simulink model "T_junction_mpc"  (R2022b)
settings: Solver=FixedStepAuto  StartTime=0.0  StopTime=293.175  FixedStep=0.025  RelTol=1e-3
values from neighbouring files (symbols this model uses):
  Aod = God.A    [mpcDesign.m]
  beta = 0.13534    [mpcDesign.m]    (also in simSysID.m)
  Bod = God.B    [mpcDesign.m]
  Cod = God.C    [mpcDesign.m]
  Dmn = Gmn.D    [mpcDesign.m]
  Dod = God.D    [mpcDesign.m]
  dt = 1/samplingRate    (= 0.025)    [plantConstants.m]    (also in sysID.m)
  eventQueue = [ ... (first row only)    [mpcDesign.m]
  forgettingFactor = 1 - dt/tau    [mpcDesign.m]
  G = idss(blkdiag(A_0, A_0),          [B_0; B_0],          blkdiag(C_0, C_0),          [D_0; D_0],          blkdiag(K_0, K_0),          x_0, dt)    [get1stOrderMdl.m]    (also in get2ndOrderMdl.m; getIntegratorMdl.m; stateEst_.m = eye(ns); stateEstimator.m = eye(ns))
  God = getoutdist(ampc)    [mpcDesign.m]
  ni = no    (= 3)    [plantConstants.m]
  no = 3    [plantConstants.m]    (also in sysID.m = length(outputs))
  np = ni + 1    [get1stOrderMdl.m]    (also in get2ndOrderMdl.m = ni + 2; getIntegratorMdl.m = ni)
  nullEv = struct('r', [0; 0; 0; 0; 0; 0], 'preT', 0, 'moveT', 0, 'postT', 0)    [mpcDesign.m]    (also in simSysID.m)
  u_max = [80; 80; 80]    [plantConstants.m]
  uwt0 = zeros(1, ni)    [mpcDesign.m]
  y_max = 612*ones(2*no, 1)    [plantConstants.m]
  ywt0 = zeros(1, 2*no)    [mpcDesign.m]    (also in simSysID.m)
undefined symbols (not defined in the file or in its folder): Discrete, lpfDen, lpfNum, N0, R0, Time, u_o, y_o
libraries: ctrlSharedLib x2, simulink_extras x1, mpclib x1
settings Model: PauseTimes=21.75  Creator=khqc  LastModifiedBy=khqc
settings DataIOCC: ExternalInput=[t, r]  OutputOption=SpecifiedOutputTimes  OutputTimes=t
settings OptimizationCC: UseDivisionForNetSlopeComputation=on  GainParamInheritBuiltInType=on  UseFloatMulNetSlope=on  StrengthReduction=on  PassReuseOutputArgsAs=Individual arguments  ZeroExternalMemoryAtStartup=off  ZeroInternalMemoryAtStartup=off  NoFixptDivByZeroProtection=on  EfficientFloat2IntCast=on  LifeSpan=1  OptimizeBlockOrder=speed  OptimizationPriority=Speed  OptimizationCustomize=off  MultiThreadedLoops=on  EfficientTunableParamExpr=on
settings DebuggingCC: ReadBeforeWriteMsg=EnableAllAsError  WriteAfterWriteMsg=EnableAllAsError  WriteAfterReadMsg=EnableAllAsError  IntegerOverflowMsg=error  ParameterTunabilityLossMsg=error  UniqueDataStoreMsg=error  BusObjectLabelMismatch=error  NonBusSignalsTreatedAsBus=error  SFInvalidInputDataAccessInChartInitDiag=error  SFTransitionOutsideNaturalParentDiag=error  SFUnreachableExecutionPathDiag=error  SFUndirectedBroadcastEventsDiag=error  IntegerSaturationMsg=error  ForceCombineOutputUpdateInSim=on
settings HardwareCC: ProdBitPerLong=64  ProdLongLongMode=on  ProdHWDeviceType=Intel->x86-64 (Linux 64)
settings ModelReferenceCC: ModelReferenceMinAlgLoopOccurrences=on
settings SFSimCC: MATLABDynamicMemAlloc=off
settings RTWCC: Description=Embedded Coder  SystemTargetFile=ert.tlc  GenCodeOnly=on  PackageGeneratedCodeAndArtifacts=on  TemplateMakefile=ert_default_tmf  GenerateReport=on  BuildConfiguration=Faster Runs  IncludeHyperlinkInReport=on  LaunchReport=on  TargetLang=C++  GenerateTraceInfo=on  GenerateTraceReport=on  GenerateTraceReportSl=on  GenerateTraceReportSf=on  GenerateTraceReportEml=on
settings CodeAppCC: ForceParamTrailComments=on  IgnoreCustomStorageClasses=off  OperatorAnnotations=on  SimulinkDataObjDesc=on  SFDataObjDesc=on  MATLABFcnDesc=on  CustomSymbolStrGlobalVar=rt$N$M  CustomSymbolStrType=$N$M  CustomSymbolStrFcn=$N$M$F  CustomSymbolStrMacro=$N$M  InsertBlockDesc=on  StateflowObjectComments=on  MATLABSourceComments=on  EnableCustomComments=on  ReqsInCode=on
settings ERTTargetCC: TargetLangStandard=C++11 (ISO)  GenerateSampleERTMain=on  CombineSignalStateStructs=on  SuppressErrorStatus=on  SupportAbsoluteTime=off  CodeInterfacePackaging=C++ class  SupportComplex=off  SupportNonInlinedSFcns=on  SupportVariableSizeSignals=on  CastingMode=Standards  RootIOFormat=Structure reference  RTWCAPIParams=on  ERTCustomFileTemplate=example_file_process.tlc  ERTFilePackagingFormat=CompactWithDataFile

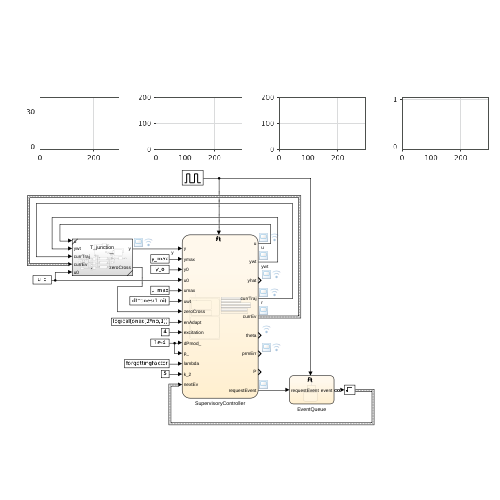
[thumbnail: Simulink's stored preview of the top-level diagram]
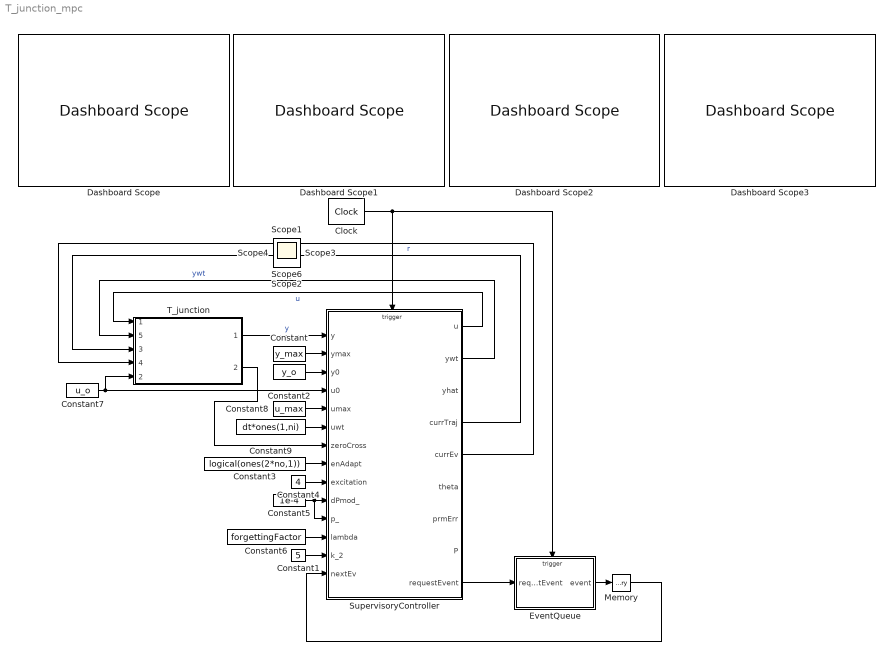
== system T_junction_mpc ==
  Clock : simulink_extras/Flip Flops/Clock  period=2*dt
  Constant : Constant  Value=y_max  VectorParams1D=off  SampleTime=-1
  Constant1 : Constant  Value=5  VectorParams1D=off  SampleTime=-1
  Constant2 : Constant  Value=y_o  VectorParams1D=off  SampleTime=-1
  Constant3 : Constant  Value=logical(ones(2*no,1))  VectorParams1D=off  SampleTime=-1
  Constant4 : Constant  Value=4  VectorParams1D=off  SampleTime=-1
  Constant5 : Constant  Value=1e-4  VectorParams1D=off  SampleTime=-1
  Constant6 : Constant  Value=forgettingFactor  VectorParams1D=off  SampleTime=-1
  Constant7 : Constant  Value=u_o  VectorParams1D=off  SampleTime=-1
  Constant8 : Constant  Value=u_max  VectorParams1D=off  SampleTime=-1
  Constant9 : Constant  Value=dt*ones(1,ni)  VectorParams1D=off  SampleTime=-1
  Dashboard Scope{,1..3} (4 alike) : DashboardScope  Ymin=0  Ymax=200
  EventQueue : Stateflow chart  TreatAsAtomicUnit=on
  Memory : Memory  InitialCondition=nullEv
  SupervisoryController : Stateflow chart  TreatAsAtomicUnit=on
  T_junction : Subsystem  ReferencedSubsystem=T_junction
      settings: PortSchema="{\"entries\":[{\"content\":{\"sides\":[{\"content\":{\"connectorIds\":[\"In1\",\"In5\",\"In3\",\"In4\",\"In2\"]},\"type\":\"ConnectorPlacement.EquallySpacedRectSide\",\"uuid\":\"0943685f-600e-41af-a665-bcc16d9a094a\"},{\"content\":{\"connectorIds\":[\"Out1\",\"Out2\"],\"side\":\"RIGHT\"},\"type\":\"ConnectorPlacement.EquallySpacedRectSide\",\"uuid\":\"88ff40b9-19c0-4ac1-b133-2a32304c8b0f\"},{\"content\":{\"connectorIds\":[],\"side\":\"TOP\"},\"type\":\"ConnectorPlacement.EquallySpacedRectSide\",\"uuid\":\"62f73c3a-6759-48ef-88af-8d02c7b37c1f\"}]},\"type\":\"ConnectorPlacement.EquallySpacedConnector\",\"uuid\":\"9de5309d-a658-4a97-a42e-d25e12f93191\"}],\"packageUris\":[\"http://schema.mathworks.com/mf0/Connector/R2020b\"],\"version\":\"1.0\"}"
  Scope{,1..4,6} (6 alike) : Scope
  wires:
  SupervisoryController/1(u) -> T_junction/1  "u"
  Clock/1 -> EventQueue/Trigger, SupervisoryController/Trigger
  Constant/1 -> SupervisoryController/2(ymax)
  Constant7/1 -> SupervisoryController/4(u0), T_junction/2
  Constant3/1 -> SupervisoryController/8(enAdapt)
  T_junction/1 -> SupervisoryController/1(y)  "y"
  Constant4/1 -> SupervisoryController/9(excitation)
  Constant2/1 -> SupervisoryController/3(y0)
  Memory/1 -> SupervisoryController/14(nextEv)
  EventQueue/1(event) -> Memory/1
  Constant5/1 -> SupervisoryController/10(dPmod_), SupervisoryController/11(p_)
  Constant6/1 -> SupervisoryController/12(lambda)
  SupervisoryController/9(requestEvent) -> EventQueue/1(requestEvent)
  SupervisoryController/5(currEv) -> T_junction/4
  SupervisoryController/4(currTraj) -> T_junction/3  "r"
  SupervisoryController/2(ywt) -> T_junction/5  "ywt"
  T_junction/2 -> SupervisoryController/7(zeroCross)
  Constant1/1 -> SupervisoryController/13(k_2)
  Constant8/1 -> SupervisoryController/5(umax)
  Constant9/1 -> SupervisoryController/6(uwt)

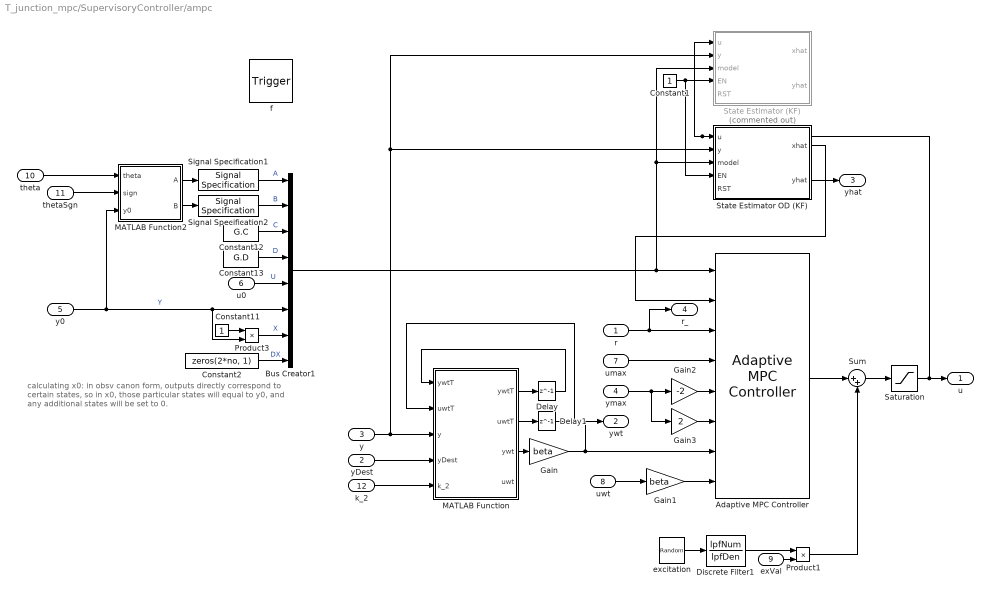
== system T_junction_mpc/SupervisoryController/ampc ==
  note: calculating x0:
      | in obsv canon form, outputs directly correspond to certain states, so in x0, those particular states will equal to y0, and any additional states will be set to 0.
  r : Inport  OutDataTypeStr=double  PortDimensions=[2*no, 1]
  yDest : Inport  Port=2  OutDataTypeStr=double  PortDimensions=[2*no, 1]
  y : Inport  Port=3  OutDataTypeStr=double  PortDimensions=[2*no, 1]
  ymax : Inport  Port=4  OutDataTypeStr=double  PortDimensions=[2*no,1]
  y0 : Inport  Port=5  OutDataTypeStr=double  PortDimensions=[2*no, 1]
  u0 : Inport  Port=6  OutDataTypeStr=double  PortDimensions=[ni, 1]
  umax : Inport  Port=7  OutDataTypeStr=double  PortDimensions=[ni, 1]
  uwt : Inport  Port=8  OutDataTypeStr=double  PortDimensions=[1, ni]
  exVal : Inport  Port=9  OutDataTypeStr=double  PortDimensions=1
  theta : Inport  Port=10  OutDataTypeStr=double  PortDimensions=[2*np*no, 1]
  thetaSgn : Inport  Port=11  OutDataTypeStr=double  PortDimensions=[2*np*no, 1]
  k_2 : Inport  Port=12  OutDataTypeStr=double  PortDimensions=1
  f : TriggerPort  TriggerType=function-call  VariantControl=(inherit)
      settings: CopyFcn=Stateflow.SLINSF.SimulinkMan.removeBlockPreDeleteFcn  PreDeleteFcn=Stateflow.SLINSF.SimulinkMan.unsafePredeleteFcn
  Adaptive MPC Controller : mpclib/Adaptive MPC Controller  SCDEnableBlockLinearizationSpecification=on  mpcobj=ampc  enable_value=0  updateMPCinCallerWorkspace=on  md_inport=off  mv_inport=off  uref_inport=off  return_cost=off  return_mvseq=off  return_qpstatus=off  return_xseq=off  return_state=off  return_ovseq=off  state_inport=on  isltv_plant=off  umin_inport=off  umax_inport=on  ymin_inport=on  ymax_inport=on  cc_inport=off  ywt_inport=on  uwt_inport=on  duwt_inport=off  rhoeps_inport=off  pm_inport=off  MaximumP=10  HorizonChoice=FixedHorizon  BlockDataType=double  SampleTimeInherited=on  switch_inport=off
  Bus Creator1 : BusCreator  Inputs=8  OutDataTypeStr=Bus: mdl_bus  NonVirtualBus=on
  Constant1 : Constant  VectorParams1D=off
  Constant11 : Constant  VectorParams1D=off
  Constant12 : Constant  Value=G.C  VectorParams1D=off
  Constant13 : Constant  Value=G.D  VectorParams1D=off
  Constant2 : Constant  Value=zeros(2*no, 1)  VectorParams1D=off
  Delay : Delay  DelayLength=1  InitialCondition=ywt0
  Delay1 : Delay  DelayLength=1  InitialCondition=uwt0
  Discrete Filter1 : DiscreteFilter  Numerator=lpfNum  Denominator=lpfDen
  Gain : Gain  Gain=beta
  Gain1 : Gain  Gain=beta
  Gain2 : Gain  Gain=-2
  Gain3 : Gain  Gain=2
  MATLAB Function : MATLAB Function  TreatAsAtomicUnit=on
  MATLAB Function2 : MATLAB Function  TreatAsAtomicUnit=on
  Product1 : Product
  Product3 : Product
  Saturation : Saturate  UpperLimit=1000  LowerLimit=0
  Signal Specification1 : SignalSpecification  Dimensions=size(G.A)
  Signal Specification2 : SignalSpecification  Dimensions=size(G.B)
  State Estimator (KF) : Subsystem  Commented=on
      settings: MinAlgLoopOccurrences=on
  State Estimator OD (KF) : Subsystem
      settings: MinAlgLoopOccurrences=on
  Sum : Sum  Inputs=|++
  excitation : RandomNumber  Mean=[0 0 0]  Variance=[1 1 1]  Seed=[12345 12346 12347]
  u : Outport
  ywt : Outport  Port=2
  yhat : Outport  Port=3
  r_ : Outport  Port=4
  wires:
  Saturation/1 -> u/1, State Estimator (KF)/1(u), State Estimator OD (KF)/1(u)
  excitation/1 -> Discrete Filter1/1
  Discrete Filter1/1 -> Product1/1
  exVal/1 -> Product1/2
  Product1/1 -> Sum/2
  Adaptive MPC Controller/1 -> Sum/1
  r/1 -> r_/1, Adaptive MPC Controller/3
  Delay/1 -> MATLAB Function/1("ywtT ")
  ymax/1 -> Gain3/1, Gain2/1
  MATLAB Function/1(ywtT) -> Delay/1
  MATLAB Function/2(uwtT) -> Delay1/1
  Delay1/1 -> MATLAB Function/2("uwtT ")
  Gain/1 -> Adaptive MPC Controller/7, ywt/1
  Gain1/1 -> Adaptive MPC Controller/8
  Sum/1 -> Saturation/1
  uwt/1 -> Gain1/1
  MATLAB Function/3(ywt) -> Gain/1
  Gain2/1 -> Adaptive MPC Controller/5
  yDest/1 -> MATLAB Function/4(yDest)
  Bus Creator1/1 -> State Estimator (KF)/3(model), State Estimator OD (KF)/3(model), Adaptive MPC Controller/1
  Product3/1 -> Bus Creator1/7  "X"
  Signal Specification1/1 -> Bus Creator1/1  "A"
  Constant11/1 -> Product3/1
  y0/1 -> MATLAB Function2/3(y0), Product3/2, Bus Creator1/6  "Y"
  Constant13/1 -> Bus Creator1/4  "D"
  Constant12/1 -> Bus Creator1/3  "C"
  MATLAB Function2/2(B) -> Signal Specification2/1
  MATLAB Function2/1(A) -> Signal Specification1/1
  Signal Specification2/1 -> Bus Creator1/2  "B"
  Constant2/1 -> Bus Creator1/8  "DX"
  thetaSgn/1 -> MATLAB Function2/2(sign)
  theta/1 -> MATLAB Function2/1(theta)
  u0/1 -> Bus Creator1/5  "U"
  Constant1/1 -> State Estimator OD (KF)/4(EN), State Estimator (KF)/4(EN)
  Gain3/1 -> Adaptive MPC Controller/6
  y/1 -> State Estimator (KF)/2(y), State Estimator OD (KF)/2(y), MATLAB Function/3(y)
  State Estimator OD (KF)/2(yhat) -> yhat/1
  State Estimator OD (KF)/1(xhat) -> Adaptive MPC Controller/2
  k_2/1 -> MATLAB Function/5(k_2)
  umax/1 -> Adaptive MPC Controller/4

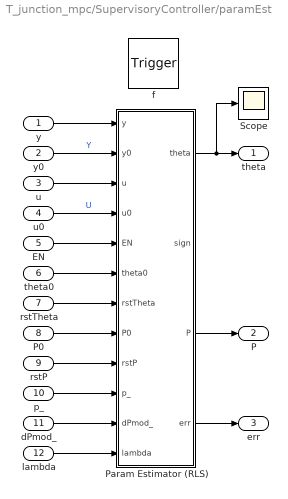
== system T_junction_mpc/SupervisoryController/paramEst ==
  y : Inport  OutDataTypeStr=double  PortDimensions=[no, 1]
  y0 : Inport  Port=2  OutDataTypeStr=double  PortDimensions=[no, 1]
  u : Inport  Port=3  OutDataTypeStr=double  PortDimensions=[ni, 1]
  u0 : Inport  Port=4  OutDataTypeStr=double  PortDimensions=[ni, 1]
  EN : Inport  Port=5  OutDataTypeStr=boolean  PortDimensions=[no, 1]
  theta0 : Inport  Port=6  OutDataTypeStr=double  PortDimensions=[np*no, 1]
  rstTheta : Inport  Port=7  OutDataTypeStr=boolean  PortDimensions=1
  P0 : Inport  Port=8  OutDataTypeStr=double  PortDimensions=[np*no, np*no]
  rstP : Inport  Port=9  OutDataTypeStr=boolean  PortDimensions=1
  p_ : Inport  Port=10  OutDataTypeStr=double  PortDimensions=1
  dPmod_ : Inport  Port=11  OutDataTypeStr=double  PortDimensions=1
  lambda : Inport  Port=12  OutDataTypeStr=double  PortDimensions=1
  f : TriggerPort  TriggerType=function-call  VariantControl=(inherit)
      settings: CopyFcn=Stateflow.SLINSF.SimulinkMan.removeBlockPreDeleteFcn  PreDeleteFcn=Stateflow.SLINSF.SimulinkMan.unsafePredeleteFcn
  Param Estimator (RLS) : Subsystem
  Scope : Scope
  theta : Outport
  P : Outport  Port=2
  err : Outport  Port=3
  wires:
  y0/1 -> Param Estimator (RLS)/2(y0)  "Y"
  u0/1 -> Param Estimator (RLS)/4(u0)  "U"
  y/1 -> Param Estimator (RLS)/1(y)
  u/1 -> Param Estimator (RLS)/3(u)
  EN/1 -> Param Estimator (RLS)/5(EN)
  theta0/1 -> Param Estimator (RLS)/6(theta0)
  rstTheta/1 -> Param Estimator (RLS)/7(rstTheta)
  P0/1 -> Param Estimator (RLS)/8(P0)
  rstP/1 -> Param Estimator (RLS)/9(rstP)
  p_/1 -> Param Estimator (RLS)/10(p_)
  dPmod_/1 -> Param Estimator (RLS)/11(dPmod_)
  lambda/1 -> Param Estimator (RLS)/12(lambda)
  Param Estimator (RLS)/1(theta) -> Scope/1, theta/1
  Param Estimator (RLS)/3(P) -> P/1
  Param Estimator (RLS)/4(err) -> err/1

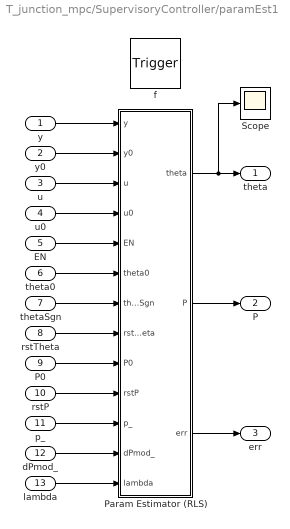
== system T_junction_mpc/SupervisoryController/paramEst1 ==
  y : Inport  OutDataTypeStr=double  PortDimensions=[no, 1]
  y0 : Inport  Port=2  OutDataTypeStr=double  PortDimensions=[no, 1]
  u : Inport  Port=3  OutDataTypeStr=double  PortDimensions=[ni, 1]
  u0 : Inport  Port=4  OutDataTypeStr=double  PortDimensions=[ni, 1]
  EN : Inport  Port=5  OutDataTypeStr=boolean  PortDimensions=[no, 1]
  theta0 : Inport  Port=6  OutDataTypeStr=double  PortDimensions=[np*no, 1]
  thetaSgn : Inport  Port=7  OutDataTypeStr=double  PortDimensions=[np*no, 1]
  rstTheta : Inport  Port=8  OutDataTypeStr=boolean  PortDimensions=1
  P0 : Inport  Port=9  OutDataTypeStr=double  PortDimensions=[np*no, np*no]
  rstP : Inport  Port=10  OutDataTypeStr=boolean  PortDimensions=1
  p_ : Inport  Port=11  OutDataTypeStr=double  PortDimensions=1
  dPmod_ : Inport  Port=12  OutDataTypeStr=double  PortDimensions=1
  lambda : Inport  Port=13  OutDataTypeStr=double  PortDimensions=1
  f : TriggerPort  TriggerType=function-call  VariantControl=(inherit)
      settings: CopyFcn=Stateflow.SLINSF.SimulinkMan.removeBlockPreDeleteFcn  PreDeleteFcn=Stateflow.SLINSF.SimulinkMan.unsafePredeleteFcn
  Param Estimator (RLS) : Subsystem
  Scope : Scope
  theta : Outport
  P : Outport  Port=2
  err : Outport  Port=3
  wires:
  y0/1 -> Param Estimator (RLS)/2(y0)
  u0/1 -> Param Estimator (RLS)/4(u0)
  y/1 -> Param Estimator (RLS)/1(y)
  u/1 -> Param Estimator (RLS)/3(u)
  EN/1 -> Param Estimator (RLS)/5(EN)
  theta0/1 -> Param Estimator (RLS)/6(theta0)
  rstTheta/1 -> Param Estimator (RLS)/8(rstTheta)
  P0/1 -> Param Estimator (RLS)/9(P0)
  rstP/1 -> Param Estimator (RLS)/10(rstP)
  p_/1 -> Param Estimator (RLS)/11(p_)
  dPmod_/1 -> Param Estimator (RLS)/12(dPmod_)
  lambda/1 -> Param Estimator (RLS)/13(lambda)
  Param Estimator (RLS)/1(theta) -> Scope/1, theta/1
  Param Estimator (RLS)/2(P) -> P/1
  Param Estimator (RLS)/3(err) -> err/1
  thetaSgn/1 -> Param Estimator (RLS)/7(thetaSgn)

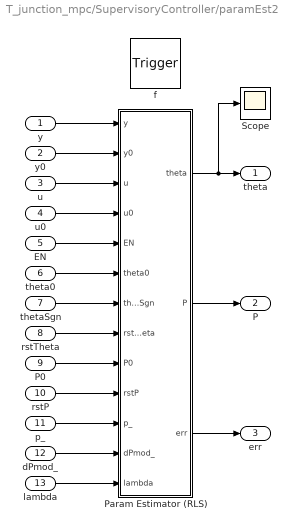
== system T_junction_mpc/SupervisoryController/paramEst2 ==
  y : Inport  OutDataTypeStr=double  PortDimensions=[no, 1]
  y0 : Inport  Port=2  OutDataTypeStr=double  PortDimensions=[no, 1]
  u : Inport  Port=3  OutDataTypeStr=double  PortDimensions=[ni, 1]
  u0 : Inport  Port=4  OutDataTypeStr=double  PortDimensions=[ni, 1]
  EN : Inport  Port=5  OutDataTypeStr=boolean  PortDimensions=[no, 1]
  theta0 : Inport  Port=6  OutDataTypeStr=double  PortDimensions=[np*no, 1]
  thetaSgn : Inport  Port=7  OutDataTypeStr=double  PortDimensions=[np*no, 1]
  rstTheta : Inport  Port=8  OutDataTypeStr=boolean  PortDimensions=1
  P0 : Inport  Port=9  OutDataTypeStr=double  PortDimensions=[np*no, np*no]
  rstP : Inport  Port=10  OutDataTypeStr=boolean  PortDimensions=1
  p_ : Inport  Port=11  OutDataTypeStr=double  PortDimensions=1
  dPmod_ : Inport  Port=12  OutDataTypeStr=double  PortDimensions=1
  lambda : Inport  Port=13  OutDataTypeStr=double  PortDimensions=1
  f : TriggerPort  TriggerType=function-call  VariantControl=(inherit)
      settings: CopyFcn=Stateflow.SLINSF.SimulinkMan.removeBlockPreDeleteFcn  PreDeleteFcn=Stateflow.SLINSF.SimulinkMan.unsafePredeleteFcn
  Param Estimator (RLS) : Subsystem
  Scope : Scope
  theta : Outport
  P : Outport  Port=2
  err : Outport  Port=3
  wires:
  y0/1 -> Param Estimator (RLS)/2(y0)
  u0/1 -> Param Estimator (RLS)/4(u0)
  y/1 -> Param Estimator (RLS)/1(y)
  u/1 -> Param Estimator (RLS)/3(u)
  EN/1 -> Param Estimator (RLS)/5(EN)
  theta0/1 -> Param Estimator (RLS)/6(theta0)
  rstTheta/1 -> Param Estimator (RLS)/8(rstTheta)
  P0/1 -> Param Estimator (RLS)/9(P0)
  rstP/1 -> Param Estimator (RLS)/10(rstP)
  p_/1 -> Param Estimator (RLS)/11(p_)
  dPmod_/1 -> Param Estimator (RLS)/12(dPmod_)
  lambda/1 -> Param Estimator (RLS)/13(lambda)
  Param Estimator (RLS)/1(theta) -> Scope/1, theta/1
  Param Estimator (RLS)/2(P) -> P/1
  Param Estimator (RLS)/3(err) -> err/1
  thetaSgn/1 -> Param Estimator (RLS)/7(thetaSgn)

== system T_junction_mpc/SupervisoryController/ampc/State Estimator (KF) ==
  u : Inport
  y : Inport  Port=2
  model : Inport  Port=3
  EN : Inport  Port=4
  RST : Inport  Port=5  PortDimensions=1
  Bus Selector : BusSelector  OutputSignals=A,B,C,D,U,Y,X,DX
  Display : Display
  Display1 : Display
  Kalman Filter2 : ctrlSharedLib/Kalman Filter  TimeDomain=Discrete-Time  UseCurrentEstimator=off  ModelSource=Input port  ModelSourceVariable=ss(0.95,1,1,0,1)  A=0.95  B=1  C=1  D=0  NumberOfStates=size(G.A,1)  NumberOfInputs=size(G.B,2)  NumberOfOutputs=size(G.C,1)  InitialEstimateSource=Dialog  X0=zeros(size(G.A,1),1)  P0=eye(size(G.A,1))  UseK=off  UseGH=off  NumberOfProcessNoiseInputs=1  G=eye(2)  TimeInvariantG=on  H=zeros(1,2)  TimeInvariantH=on  Q=Q0  TimeInvariantQ=off  R=R0  TimeInvariantR=off  N=N0  TimeInvariantN=off  AddInputPort=on  AddEnablePort=on  ExternalReset=Level  OutputEstimatedY=on  OutputP=off  Ts=-1
  MATLAB Function : MATLAB Function  TreatAsAtomicUnit=on
  Sum1 : Sum  Inputs=|+-
  Sum2 : Sum  Inputs=|++
  Sum3 : Sum  Inputs=|++
  Sum6 : Sum  Inputs=|+-
  xhat : Outport
  yhat : Outport  Port=2
  wires:
  Kalman Filter2/1 -> Sum2/1
  MATLAB Function/5(Q) -> Kalman Filter2/9
  MATLAB Function/2(B) -> Display1/1, Kalman Filter2/6
  RST/1 -> Kalman Filter2/4
  MATLAB Function/1(A) -> Display/1, Kalman Filter2/5
  model/1 -> Bus Selector/1
  Bus Selector/7 -> Sum2/2  "<X>"
  MATLAB Function/3(C) -> Kalman Filter2/7
  Bus Selector/1 -> MATLAB Function/1(Ap)  "<A>"
  Bus Selector/2 -> MATLAB Function/2(Bp)  "<B>"
  MATLAB Function/4(D) -> Kalman Filter2/8
  EN/1 -> Kalman Filter2/3
  Bus Selector/3 -> MATLAB Function/3(Cp)  "<C>"
  Bus Selector/4 -> MATLAB Function/4(Dp)  "<D>"
  Bus Selector/5 -> Sum1/2  "<U>"
  Sum2/1 -> xhat/1
  Bus Selector/6 -> Sum3/2, Sum6/2  "<Y>"
  y/1 -> Sum6/1
  MATLAB Function/6(R) -> Kalman Filter2/10
  MATLAB Function/7(N) -> Kalman Filter2/11
  u/1 -> Sum1/1
  Sum1/1 -> Kalman Filter2/1
  Sum6/1 -> Kalman Filter2/2
  Kalman Filter2/2 -> Sum3/1
  Sum3/1 -> yhat/1

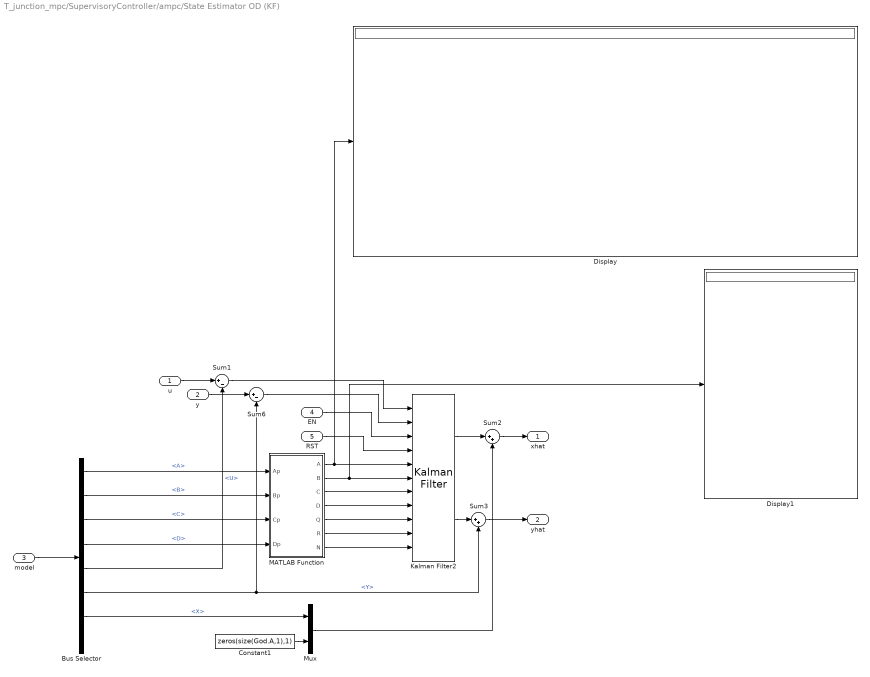
== system T_junction_mpc/SupervisoryController/ampc/State Estimator OD (KF) ==
  u : Inport
  y : Inport  Port=2
  model : Inport  Port=3
  EN : Inport  Port=4
  RST : Inport  Port=5  PortDimensions=1
  Bus Selector : BusSelector  OutputSignals=A,B,C,D,U,Y,X,DX
  Constant1 : Constant  Value=zeros(size(God.A,1),1)  VectorParams1D=off
  Display : Display
  Display1 : Display
  Kalman Filter2 : ctrlSharedLib/Kalman Filter  TimeDomain=Discrete-Time  UseCurrentEstimator=off  ModelSource=Input port  ModelSourceVariable=ss(0.95,1,1,0,1)  A=0.95  B=1  C=1  D=0  NumberOfStates=size(G.A,1) + size(God.A,1)  NumberOfInputs=size(G.B,2)  NumberOfOutputs=size(G.C,1)  InitialEstimateSource=Dialog  X0=zeros(size(G.A,1) + size(God.A,1),1)  P0=eye(size(G.A,1) + size(God.A,1))  UseK=off  UseGH=off  NumberOfProcessNoiseInputs=1  G=eye(2)  TimeInvariantG=on  H=zeros(1,2)  TimeInvariantH=on  Q=Q0  TimeInvariantQ=off  R=R0  TimeInvariantR=off  N=N0  TimeInvariantN=off  AddInputPort=on  AddEnablePort=on  ExternalReset=Level  OutputEstimatedY=on  OutputP=off  Ts=-1
  MATLAB Function : MATLAB Function  TreatAsAtomicUnit=on
  Mux : Mux  Inputs=2
  Sum1 : Sum  Inputs=|+-
  Sum2 : Sum  Inputs=|++
  Sum3 : Sum  Inputs=|++
  Sum6 : Sum  Inputs=|+-
  xhat : Outport
  yhat : Outport  Port=2
  wires:
  Kalman Filter2/1 -> Sum2/1
  MATLAB Function/5(Q) -> Kalman Filter2/9
  MATLAB Function/2(B) -> Display1/1, Kalman Filter2/6
  RST/1 -> Kalman Filter2/4
  MATLAB Function/1(A) -> Display/1, Kalman Filter2/5
  model/1 -> Bus Selector/1
  Bus Selector/7 -> Mux/1  "<X>"
  MATLAB Function/3(C) -> Kalman Filter2/7
  Bus Selector/1 -> MATLAB Function/1(Ap)  "<A>"
  Bus Selector/2 -> MATLAB Function/2(Bp)  "<B>"
  MATLAB Function/4(D) -> Kalman Filter2/8
  EN/1 -> Kalman Filter2/3
  Bus Selector/3 -> MATLAB Function/3(Cp)  "<C>"
  Bus Selector/4 -> MATLAB Function/4(Dp)  "<D>"
  Constant1/1 -> Mux/2
  Bus Selector/5 -> Sum1/2  "<U>"
  Sum2/1 -> xhat/1
  Bus Selector/6 -> Sum3/2, Sum6/2  "<Y>"
  y/1 -> Sum6/1
  MATLAB Function/6(R) -> Kalman Filter2/10
  MATLAB Function/7(N) -> Kalman Filter2/11
  u/1 -> Sum1/1
  Sum1/1 -> Kalman Filter2/1
  Sum6/1 -> Kalman Filter2/2
  Kalman Filter2/2 -> Sum3/1
  Sum3/1 -> yhat/1
  Mux/1 -> Sum2/2

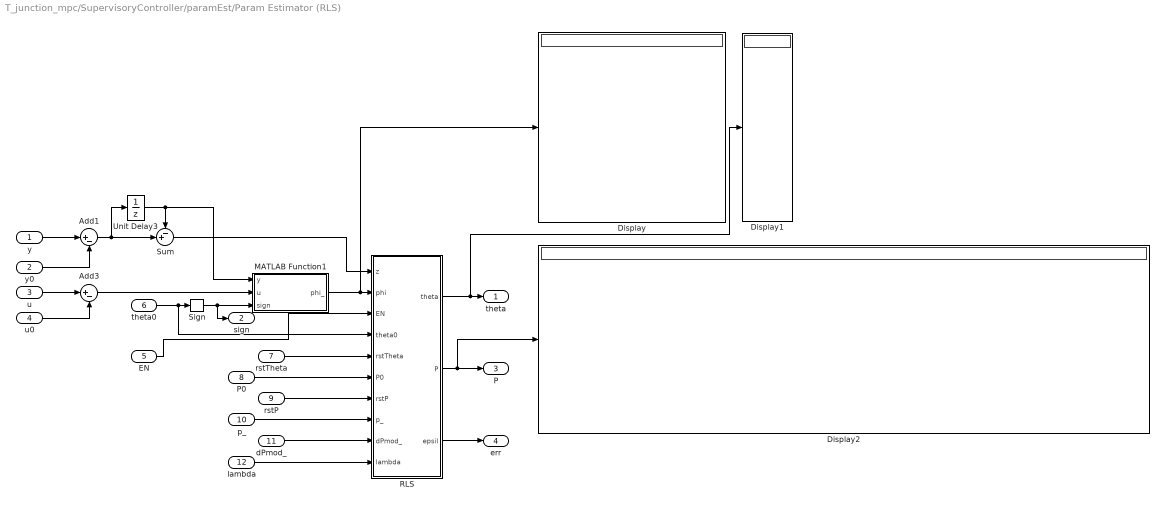
== system T_junction_mpc/SupervisoryController/paramEst/Param Estimator (RLS) ==
  y : Inport
  y0 : Inport  Port=2
  u : Inport  Port=3
  u0 : Inport  Port=4
  EN : Inport  Port=5
  theta0 : Inport  Port=6
  rstTheta : Inport  Port=7
  P0 : Inport  Port=8
  rstP : Inport  Port=9
  p_ : Inport  Port=10
  dPmod_ : Inport  Port=11
  lambda : Inport  Port=12
  Add1 : Sum  Inputs=|+-
  Add3 : Sum  Inputs=|+-
  Display : Display
  Display1 : Display
  Display2 : Display
  MATLAB Function1 : MATLAB Function  TreatAsAtomicUnit=on
  RLS : Subsystem
  Sign : Signum
  Sum : Sum  Inputs=-+|
  Unit Delay3 : UnitDelay  SampleTime=-1  HasFrameUpgradeWarning=on
  theta : Outport
  sign : Outport  Port=2
  P : Outport  Port=3
  err : Outport  Port=4
  wires:
  p_/1 -> RLS/8(p_)
  P0/1 -> RLS/6(P0)
  RLS/3(epsil) -> err/1
  u/1 -> Add3/1
  Sign/1 -> sign/1, MATLAB Function1/3(sign)
  Sum/1 -> RLS/1(z)
  rstTheta/1 -> RLS/5(rstTheta)
  Add1/1 -> Sum/2, Unit Delay3/1
  y0/1 -> Add1/2
  theta0/1 -> RLS/4(theta0), Sign/1
  y/1 -> Add1/1
  dPmod_/1 -> RLS/9(dPmod_)
  Add3/1 -> MATLAB Function1/2(u)
  Unit Delay3/1 -> MATLAB Function1/1(y), Sum/1
  RLS/1(theta) -> theta/1, Display1/1
  lambda/1 -> RLS/10(lambda)
  rstP/1 -> RLS/7(rstP)
  RLS/2(P) -> P/1, Display2/1
  MATLAB Function1/1(phi_) -> Display/1, RLS/2(phi)
  u0/1 -> Add3/2
  EN/1 -> RLS/3(EN)

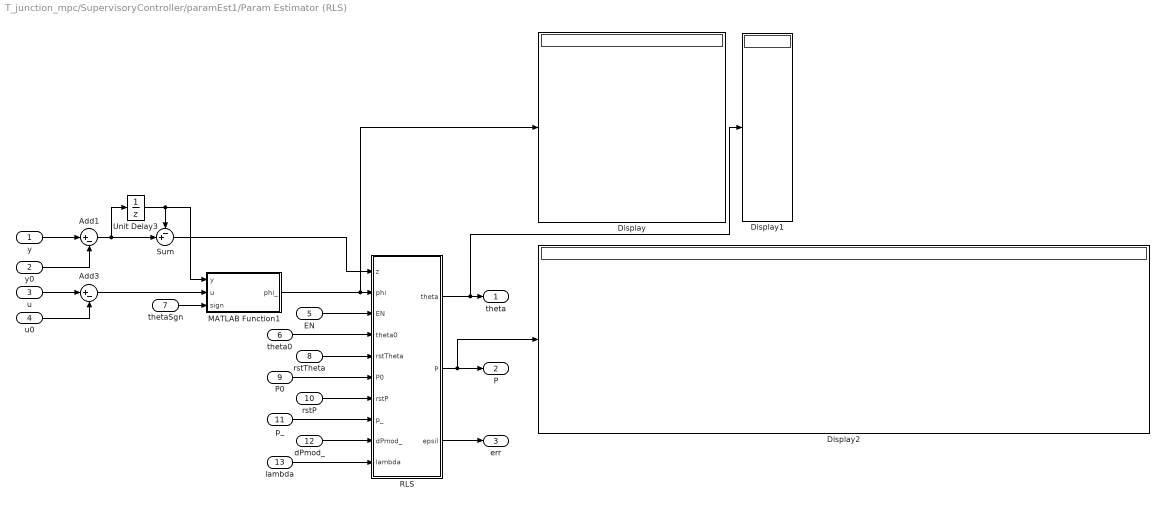
== system T_junction_mpc/SupervisoryController/paramEst1/Param Estimator (RLS) ==
  y : Inport
  y0 : Inport  Port=2
  u : Inport  Port=3
  u0 : Inport  Port=4
  EN : Inport  Port=5
  theta0 : Inport  Port=6
  thetaSgn : Inport  Port=7
  rstTheta : Inport  Port=8
  P0 : Inport  Port=9
  rstP : Inport  Port=10
  p_ : Inport  Port=11
  dPmod_ : Inport  Port=12
  lambda : Inport  Port=13
  Add1 : Sum  Inputs=|+-
  Add3 : Sum  Inputs=|+-
  Display : Display
  Display1 : Display
  Display2 : Display
  MATLAB Function1 : MATLAB Function  TreatAsAtomicUnit=on
  RLS : Subsystem
  Sum : Sum  Inputs=-+|
  Unit Delay3 : UnitDelay  SampleTime=-1  HasFrameUpgradeWarning=on
  theta : Outport
  P : Outport  Port=2
  err : Outport  Port=3
  wires:
  p_/1 -> RLS/8(p_)
  P0/1 -> RLS/6(P0)
  RLS/3(epsil) -> err/1
  u/1 -> Add3/1
  thetaSgn/1 -> MATLAB Function1/3(sign)
  Sum/1 -> RLS/1(z)
  rstTheta/1 -> RLS/5(rstTheta)
  Add1/1 -> Sum/2, Unit Delay3/1
  y0/1 -> Add1/2
  theta0/1 -> RLS/4(theta0)
  y/1 -> Add1/1
  dPmod_/1 -> RLS/9(dPmod_)
  Add3/1 -> MATLAB Function1/2(u)
  Unit Delay3/1 -> MATLAB Function1/1(y), Sum/1
  RLS/1(theta) -> theta/1, Display1/1
  lambda/1 -> RLS/10(lambda)
  rstP/1 -> RLS/7(rstP)
  RLS/2(P) -> P/1, Display2/1
  MATLAB Function1/1(phi_) -> Display/1, RLS/2(phi)
  u0/1 -> Add3/2
  EN/1 -> RLS/3(EN)

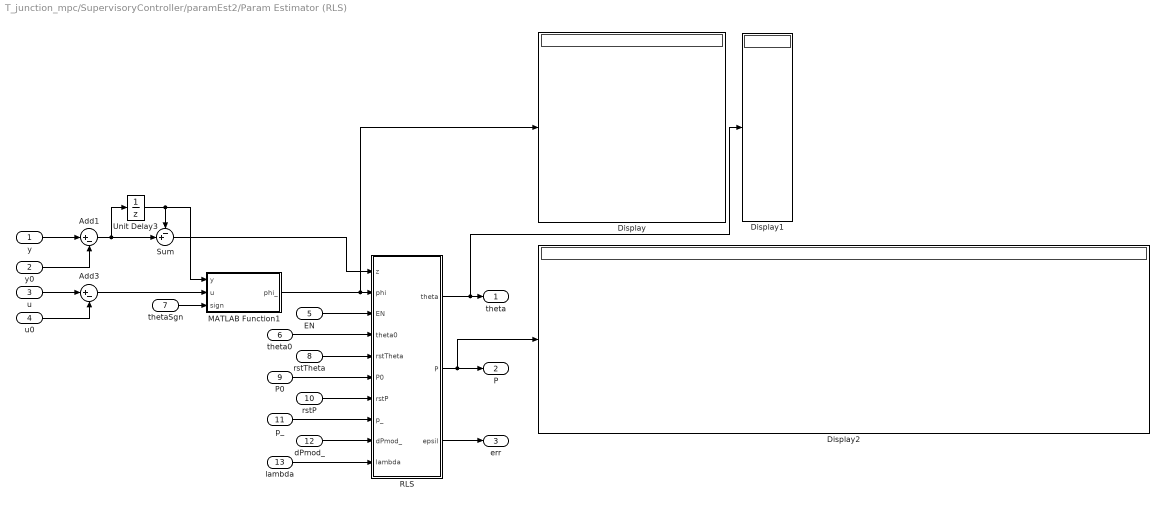
== system T_junction_mpc/SupervisoryController/paramEst2/Param Estimator (RLS) ==
  y : Inport
  y0 : Inport  Port=2
  u : Inport  Port=3
  u0 : Inport  Port=4
  EN : Inport  Port=5
  theta0 : Inport  Port=6
  thetaSgn : Inport  Port=7
  rstTheta : Inport  Port=8
  P0 : Inport  Port=9
  rstP : Inport  Port=10
  p_ : Inport  Port=11
  dPmod_ : Inport  Port=12
  lambda : Inport  Port=13
  Add1 : Sum  Inputs=|+-
  Add3 : Sum  Inputs=|+-
  Display : Display
  Display1 : Display
  Display2 : Display
  MATLAB Function1 : MATLAB Function  TreatAsAtomicUnit=on
  RLS : Subsystem
  Sum : Sum  Inputs=-+|
  Unit Delay3 : UnitDelay  SampleTime=-1  HasFrameUpgradeWarning=on
  theta : Outport
  P : Outport  Port=2
  err : Outport  Port=3
  wires:
  p_/1 -> RLS/8(p_)
  P0/1 -> RLS/6(P0)
  RLS/3(epsil) -> err/1
  u/1 -> Add3/1
  thetaSgn/1 -> MATLAB Function1/3(sign)
  Sum/1 -> RLS/1(z)
  rstTheta/1 -> RLS/5(rstTheta)
  Add1/1 -> Sum/2, Unit Delay3/1
  y0/1 -> Add1/2
  theta0/1 -> RLS/4(theta0)
  y/1 -> Add1/1
  dPmod_/1 -> RLS/9(dPmod_)
  Add3/1 -> MATLAB Function1/2(u)
  Unit Delay3/1 -> MATLAB Function1/1(y), Sum/1
  RLS/1(theta) -> theta/1, Display1/1
  lambda/1 -> RLS/10(lambda)
  rstP/1 -> RLS/7(rstP)
  RLS/2(P) -> P/1, Display2/1
  MATLAB Function1/1(phi_) -> Display/1, RLS/2(phi)
  u0/1 -> Add3/2
  EN/1 -> RLS/3(EN)

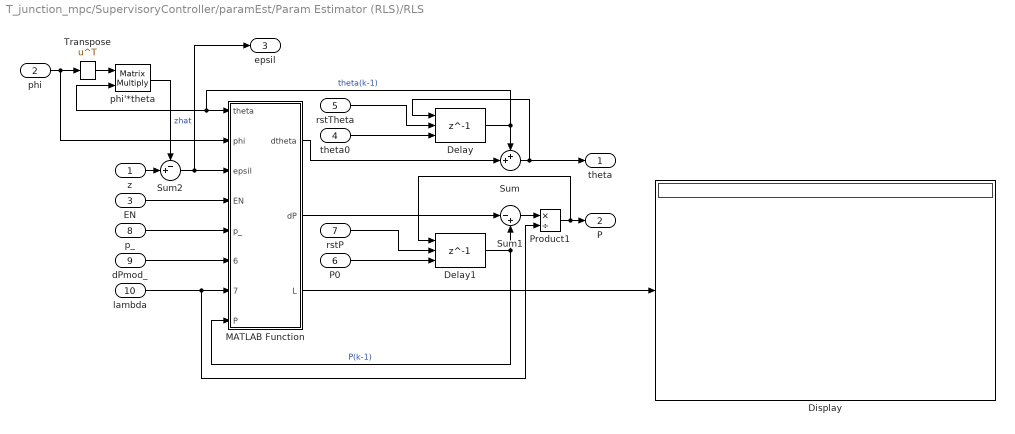
== system T_junction_mpc/SupervisoryController/paramEst/Param Estimator (RLS)/RLS ==
  z : Inport
  phi : Inport  Port=2
  EN : Inport  Port=3
  theta0 : Inport  Port=4
  rstTheta : Inport  Port=5
  P0 : Inport  Port=6
  rstP : Inport  Port=7
  p_ : Inport  Port=8
  dPmod_ : Inport  Port=9
  lambda : Inport  Port=10
  Delay : Delay  DelayLength=1  InitialConditionSource=Input port  ExternalReset=Rising
      settings: InputPortMap=u0,r5,p4
  Delay1 : Delay  DelayLength=1  InitialConditionSource=Input port  ExternalReset=Rising
      settings: InputPortMap=u0,r5,p4
  Display : Display
  MATLAB Function : MATLAB Function  TreatAsAtomicUnit=on
  Product1 : Product  Inputs=*/
  Sum : Sum  Inputs=++|
  Sum1 : Sum  Inputs=|-+
  Sum2 : Sum  Inputs=-+|
  Transpose : Math  Operator=transpose
  phi'*theta : Product  Multiplication=Matrix(*)
  theta : Outport
  P : Outport  Port=2
  epsil : Outport  Port=3
  wires:
  phi/1 -> MATLAB Function/2(phi), Transpose/1
  EN/1 -> MATLAB Function/4(EN)
  P0/1 -> Delay1/3
  MATLAB Function/1(dtheta) -> Sum/2
  Delay/1 -> Sum/1, phi'*theta/2, MATLAB Function/1(theta)  "theta(k-1)"
  Sum/1 -> theta/1, Delay/1
  MATLAB Function/2(dP) -> Sum1/1
  Sum1/1 -> Product1/1
  Delay1/1 -> Sum1/2, MATLAB Function/8(P)  "P(k-1)"
  Product1/1 -> Delay1/1, P/1
  z/1 -> Sum2/2
  Transpose/1 -> phi'*theta/1
  phi'*theta/1 -> Sum2/1  "zhat"
  Sum2/1 -> epsil/1, MATLAB Function/3(epsil)
  theta0/1 -> Delay/3
  dPmod_/1 -> MATLAB Function/6(dPmod_)
  p_/1 -> MATLAB Function/5(p_)
  rstTheta/1 -> Delay/2
  rstP/1 -> Delay1/2
  lambda/1 -> Product1/2, MATLAB Function/7(lambda)
  MATLAB Function/3(L) -> Display/1

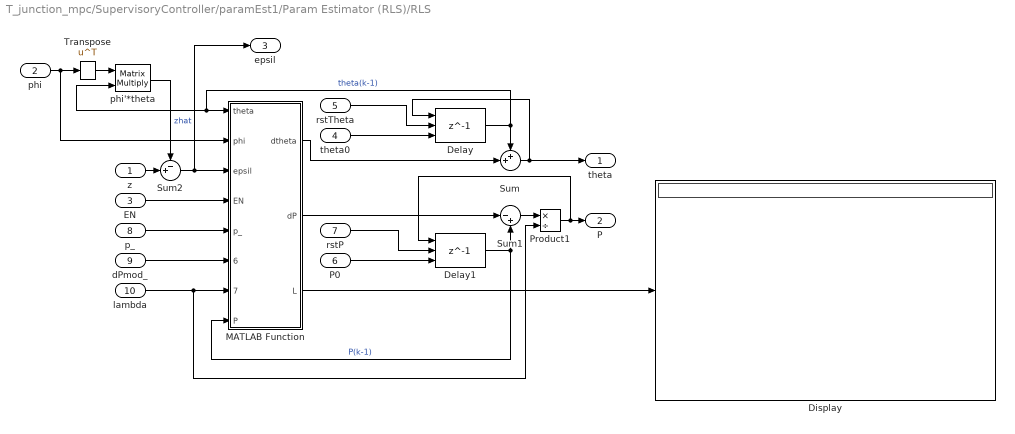
== system T_junction_mpc/SupervisoryController/paramEst1/Param Estimator (RLS)/RLS ==
  z : Inport
  phi : Inport  Port=2
  EN : Inport  Port=3
  theta0 : Inport  Port=4
  rstTheta : Inport  Port=5
  P0 : Inport  Port=6
  rstP : Inport  Port=7
  p_ : Inport  Port=8
  dPmod_ : Inport  Port=9
  lambda : Inport  Port=10
  Delay : Delay  DelayLength=1  InitialConditionSource=Input port  ExternalReset=Rising
      settings: InputPortMap=u0,r5,p4
  Delay1 : Delay  DelayLength=1  InitialConditionSource=Input port  ExternalReset=Rising
      settings: InputPortMap=u0,r5,p4
  Display : Display
  MATLAB Function : MATLAB Function  TreatAsAtomicUnit=on
  Product1 : Product  Inputs=*/
  Sum : Sum  Inputs=++|
  Sum1 : Sum  Inputs=|-+
  Sum2 : Sum  Inputs=-+|
  Transpose : Math  Operator=transpose
  phi'*theta : Product  Multiplication=Matrix(*)
  theta : Outport
  P : Outport  Port=2
  epsil : Outport  Port=3
  wires:
  phi/1 -> MATLAB Function/2(phi), Transpose/1
  EN/1 -> MATLAB Function/4(EN)
  P0/1 -> Delay1/3
  MATLAB Function/1(dtheta) -> Sum/2
  Delay/1 -> Sum/1, phi'*theta/2, MATLAB Function/1(theta)  "theta(k-1)"
  Sum/1 -> theta/1, Delay/1
  MATLAB Function/2(dP) -> Sum1/1
  Sum1/1 -> Product1/1
  Delay1/1 -> Sum1/2, MATLAB Function/8(P)  "P(k-1)"
  Product1/1 -> Delay1/1, P/1
  z/1 -> Sum2/2
  Transpose/1 -> phi'*theta/1
  phi'*theta/1 -> Sum2/1  "zhat"
  Sum2/1 -> epsil/1, MATLAB Function/3(epsil)
  theta0/1 -> Delay/3
  dPmod_/1 -> MATLAB Function/6(dPmod_)
  p_/1 -> MATLAB Function/5(p_)
  rstTheta/1 -> Delay/2
  rstP/1 -> Delay1/2
  lambda/1 -> MATLAB Function/7(lambda), Product1/2
  MATLAB Function/3(L) -> Display/1

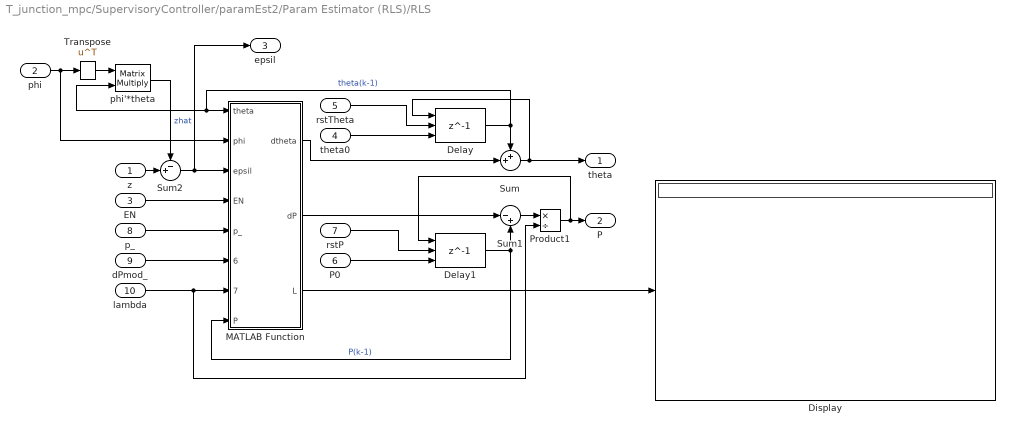
== system T_junction_mpc/SupervisoryController/paramEst2/Param Estimator (RLS)/RLS ==
  z : Inport
  phi : Inport  Port=2
  EN : Inport  Port=3
  theta0 : Inport  Port=4
  rstTheta : Inport  Port=5
  P0 : Inport  Port=6
  rstP : Inport  Port=7
  p_ : Inport  Port=8
  dPmod_ : Inport  Port=9
  lambda : Inport  Port=10
  Delay : Delay  DelayLength=1  InitialConditionSource=Input port  ExternalReset=Rising
      settings: InputPortMap=u0,r5,p4
  Delay1 : Delay  DelayLength=1  InitialConditionSource=Input port  ExternalReset=Rising
      settings: InputPortMap=u0,r5,p4
  Display : Display
  MATLAB Function : MATLAB Function  TreatAsAtomicUnit=on
  Product1 : Product  Inputs=*/
  Sum : Sum  Inputs=++|
  Sum1 : Sum  Inputs=|-+
  Sum2 : Sum  Inputs=-+|
  Transpose : Math  Operator=transpose
  phi'*theta : Product  Multiplication=Matrix(*)
  theta : Outport
  P : Outport  Port=2
  epsil : Outport  Port=3
  wires:
  phi/1 -> MATLAB Function/2(phi), Transpose/1
  EN/1 -> MATLAB Function/4(EN)
  P0/1 -> Delay1/3
  MATLAB Function/1(dtheta) -> Sum/2
  Delay/1 -> Sum/1, phi'*theta/2, MATLAB Function/1(theta)  "theta(k-1)"
  Sum/1 -> theta/1, Delay/1
  MATLAB Function/2(dP) -> Sum1/1
  Sum1/1 -> Product1/1
  Delay1/1 -> Sum1/2, MATLAB Function/8(P)  "P(k-1)"
  Product1/1 -> Delay1/1, P/1
  z/1 -> Sum2/2
  Transpose/1 -> phi'*theta/1
  phi'*theta/1 -> Sum2/1  "zhat"
  Sum2/1 -> epsil/1, MATLAB Function/3(epsil)
  theta0/1 -> Delay/3
  dPmod_/1 -> MATLAB Function/6(dPmod_)
  p_/1 -> MATLAB Function/5(p_)
  rstTheta/1 -> Delay/2
  rstP/1 -> Delay1/2
  lambda/1 -> MATLAB Function/7(lambda), Product1/2
  MATLAB Function/3(L) -> Display/1

== matlab function T_junction_mpc/SupervisoryController/paramEst/Param Estimator (RLS)/MATLAB Function1 ==
  data: y input; u input; phi_ output; sign input
function phi_ = toPhi(y, u, sign)
phi_ = toPhi_(y, u, sign);

== stateflow chart T_junction_mpc/EventQueue ==
  settings: sampleTime=dt  executeAtInitialization=1
  state idle
    event = nullEv;
  state pushEvent
    en:
    if idx <= size(eventQueue, 1)
    event = eventQueue(idx);
    disp("sending event");
    idx = idx+ 1;
    end
  (default) -> idle : {idx = 1;}
  pushEvent -> idle
  idle -> pushEvent : [requestEvent]
  data: idx local; eventQueue parameter; requestEvent input; event output Bus: event_bus; nullEv parameter
  events: measAvail input EITHER_EDGE_EVENT

== matlab function T_junction_mpc/SupervisoryController/paramEst/Param Estimator (RLS)/RLS/MATLAB Function ==
  data: theta input; phi input; epsil input; EN input; p_ input; dPmod_ input; lambda input; dtheta output; P input; dP output; L output
function [dtheta, dP, L] = rls(theta, phi, epsil, EN, p_, dPmod_, lambda, P)
[dtheta, dP, L] = rls_(theta, phi, epsil, EN, p_, dPmod_, lambda, P);

== matlab function T_junction_mpc/SupervisoryController/ampc/State Estimator OD (KF)/MATLAB Function ==
  data: Ap input; Bp input; Cp input; Dp input; A output; B output; C output; D output; Q output; R output; N output; Aod parameter; Bod parameter; Cod parameter; Dod parameter; Dmn parameter; no parameter; ni parameter
function [A, B, C, D, Q, R, N] = stateEst(Ap, Bp, Cp, Dp, Aod, Bod, Cod, Dod, Dmn, no, ni)
[A, B, C, D, Q, R, N] = stateEstimator(Ap, Bp, Cp, Dp, Aod, Bod, Cod, Dod, Dmn, no, ni);
end

== matlab function T_junction_mpc/SupervisoryController/ampc/State Estimator (KF)/MATLAB Function ==
  data: Ap input; Bp input; Cp input; Dp input; A output; B output; C output; D output; Q output; R output; N output; Dmn parameter
function [A, B, C, D, Q, R, N] = stateEst(Ap, Bp, Cp, Dp, Dmn)
[A, B, C, D, Q, R, N] = stateEst_(Ap, Bp, Cp, Dp, Dmn);
end

== matlab function T_junction_mpc/SupervisoryController/ampc/MATLAB Function ==
  data: ywtT input; uwtT input; ywtT output; uwtT output; y input; yDest input; ywt output; uwt output; dt parameter; no parameter; ni parameter; k_2 input
function [ywtT, uwtT, ywt, uwt] = wtMod(ywtT, uwtT, y, yDest, dt, no, ni, k_2)
[ywt, ywtT, uwt, uwtT] = wtMod_(y, yDest, ywtT, uwtT, dt, no, ni, k_2);

== matlab function T_junction_mpc/SupervisoryController/ampc/MATLAB Function2 ==
  data: theta input; sign input; A output; B output; y0 input; no parameter; np parameter
function [A, B] = theta2ss(theta, sign, y0, no, np)
[A, B] = theta2ss_(theta, sign, y0, no, np);

== matlab function T_junction_mpc/SupervisoryController/paramEst1/Param Estimator (RLS)/MATLAB Function1 ==
  data: y input; u input; phi_ output; sign input; no parameter; ni parameter; np parameter
function phi_ = toPhi(y, u, sign, no, ni, np)
phi_ = toPhi_(y, u, sign, no, ni, np);

== stateflow chart T_junction_mpc/SupervisoryController ==
  state Supervisor
    state EventHandler [parallel]
      settings: executionOrder=1
      state RequestEvent
        en:
        evDone = false;
        if waypt == 1 % hold curr pos
        traj(:, waypt) = y;
        else % hold last waypoint pos
        traj(:,1) = traj(:, waypt);
        waypt = 1;
        end
        requestEvent = true; % request new event
        ex:
        requestEvent = false;
      state HandleEvent
        en:
        currEv = nextEv;
        [traj, trajSize] = trajGen(currEv, y);
        disp("received event");
        du:
        [evDone, waypt, currEv.postT] = handleEvent(currEv, currEv.postT);
      (default) -> RequestEvent
      HandleEvent -> RequestEvent : [evDone]
      RequestEvent -> HandleEvent : [~isequal(nextEv, nullEv)]{evDone = false;}
    state ControlLaw [parallel]
      du:
      if any(currEv.r(1:no)) && any(zeroCross(no+1:2*no))
      rstP2 = true; rstTheta2 = true; enAdapt_(no+1:2*no) = false;
      P0_2 = P(1:np*no, 1:np*no); theta0_2 = theta(1:np*no);
      else
      rstP2 = false; rstTheta2 = false; enAdapt_(no+1:2*no) = true;
      end
      if any(currEv.r(no+1:2*no)) && any(zeroCross(1:no))
      rstP1 = true; rstTheta1 = true; enAdapt_(1:no) = false;
      P0_1 = P(np*no+1:2*np*no, np*no+1:2*np*no); theta0_1 = theta(np*no+1:2*np*no);
      else
      rstP1 = false; rstTheta1 = false; enAdapt_(1:no) = true;
      end
      [theta(1:np*no), P(1:np*no, 1:np*no), prmErr(1:no)] = ...
      paramEst1(y(1:no), y0(1:no), u, u0,...
      enAdapt_(1:no),...
      theta0_1, thetaSgn(1:np*no), rstTheta1, P0_1, rstP1,...
      p_, dPmod_, lambda);
      [theta(np*no+1:2*np*no), P(np*no+1:2*np*no, np*no+1:2*np*no), prmErr(no+1:2*no)] = ...
      paramEst2(y(no+1:2*no), y0(no+1:2*no), u, u0,...
      enAdapt_(no+1:2*no),...
      theta0_2, thetaSgn(np*no+1:2*np*no), rstTheta2, P0_2, rstP2,...
      p_, dPmod_, lambda);
      [u, ywt, yhat, currTraj] = ...
      ampc(traj(:,waypt), currEv.r, y, ymax, y0, u0, umax, uwt, excitation, theta, thetaSgn, k_2);
      settings: executionOrder=2
  state [theta,P,err] = paramEst1(y,y0,u,u0,EN,theta0,thetaSgn,rstTheta,P0,rstP,p_,dPmod_,lambda) [function]
  state [theta,P,err] = paramEst2(y,y0,u,u0,EN,theta0,thetaSgn,rstTheta,P0,rstP,p_,dPmod_,lambda) [function]
  state [u,ywt,yhat,r_] = ampc(r,yDest,y,ymax,y0,u0,umax,uwt,exVal,theta,thetaSgn,k_2) [function]
  state [theta,P,err] = paramEst(y,y0,u,u0,EN,theta0,rstTheta,P0,rstP,p_,dPmod_,lambda) [function] [commented out]
  (default) -> Supervisor : {currEv = nullEv;}
  data: event function_input; eventDone function_output; waypt_ function_output; holdT function_output; holdT function_input; event function_input; trajectory function_output; trajectorySize function_output; y_ function_input; y function_input double size=[no, 1]; y0 function_input double size=[no, 1]; u function_input double size=[ni, 1]; u0 function_input double size=[ni, 1]; EN function_input boolean size=[no, 1]; theta0 function_input double size=[np*no, 1]; thetaSgn function_input double size=[np*no, 1]; rstTheta function_input boolean size=1; P0 function_input double size=[np*no, np*no]; rstP function_input boolean size=1; p_ function_input double size=1; dPmod_ function_input double size=1; lambda function_input double size=1; theta function_output; P function_output; err function_output; y function_input double size=[no, 1]; y0 function_input double size=[no, 1]; u function_input double size=[ni, 1]; u0 function_input double size=[ni, 1]; EN function_input boolean size=[no, 1]; theta0 function_input double size=[np*no, 1]; thetaSgn function_input double size=[np*no, 1]; rstTheta function_input boolean size=1; P0 function_input double size=[np*no, np*no]; rstP function_input boolean size=1; p_ function_input double size=1; dPmod_ function_input double size=1; lambda function_input double size=1; theta function_output; P function_output; err function_output; r function_input double size=[2*no, 1]; yDest function_input double size=[2*no, 1]; y function_input double size=[2*no, 1]; ymax function_input double size=[2*no,1]; y0 function_input double size=[2*no, 1]; u0 function_input double size=[ni, 1]; umax function_input double size=[ni, 1]; uwt function_input double size=[1, ni]; exVal function_input double size=1; u function_output; ywt function_output; yhat function_output; r_ function_output; theta function_input double size=[2*np*no, 1]; thetaSgn function_input double size=[2*np*no, 1]; k_2 function_input double size=1; y function_input double size=1; y0 function_input double size=1; u function_input double size=1; u0 function_input double size=1; EN function_input double size=1; theta0 function_input double size=1; rstTheta function_input double size=1; P0 function_input double size=1; rstP function_input double size=1; p_ function_input double size=1; dPmod_ function_input double size=1; lambda function_input double size=1; theta function_output double size=1; P function_output double size=1; err function_output double size=1; u output double size=[ni, 1] =zeros(ni,1); y input double size=[2*no, 1]; ywt output double size=[1, 2*no] =ywt0; yhat output double size=[2*no, 1] =zeros(2*no,1); evDone local boolean size=1; waypt local uint16 size=1 =cast(1, 'uint16'); traj local double size=[2*no, 2400] =zeros(2*no, 2400); dt parameter double size=1; currTraj output double size=[2*no, 1] =zeros(2*no,1); currEv output Bus: event_bus size=1; ymax input double size=[2*no, 1]; y0 input double size=[2*no, 1]; u0 input double size=[ni, 1]; umax input double size=[ni, 1]; uwt input double size=[1, ni]; zeroCross input boolean size=[2*no, 1]; enAdapt input boolean size=[2*no, 1]; nullEv parameter Bus: event_bus; excitation input double size=1; theta output double size=[2*np*no, 1] =theta0; prmErr output double size=[2*no, 1]; dPmod_ input double size=1; p_ input double size=1; lambda input double size=1; k_2 input double size=1; P output double size=[2*np*no, 2*np*no] =P_0; requestEvent output boolean size=1 =false; nextEv input Bus: event_bus; trajSize local uint16 size=1 =cast(2400, 'uint16'); no parameter; np parameter; rstP1 local; rstP2 local; rstTheta1 local; rstTheta2 local; P0_1 local =P_0(1:np*no, 1:np*no); P0_2 local =P_0(np*no+1:2*np*no, np*no+1:2*np*no); theta0_1 local =theta0(1:np*no); theta0_2 local =theta0(np*no+1:2*np*no); thetaSgn local =sign(theta0); enAdapt_ local boolean size=[2*no, 1]
  events: measAvail input EITHER_EDGE_EVENT
  function [eventDone, waypt_, holdT] = handleEvent(event, holdT):
    | function [eventDone, waypt_, holdT] = handleEvent(event, holdT)
    | [eventDone, waypt_, holdT] = handleEvent_(event, waypt, holdT, y, ymax, trajSize, dt);
  function [trajectory, trajectorySize] = trajGen(event, y_):
    | function [trajectory, trajectorySize] = trajGen(event, y_)
    | [trajectory, trajectorySize] = trajGen_(event, y_, ymax, dt, no);

== matlab function T_junction_mpc/SupervisoryController/paramEst2/Param Estimator (RLS)/MATLAB Function1 ==
  data: y input; u input; phi_ output; sign input; no parameter; ni parameter; np parameter
function phi_ = toPhi(y, u, sign, no, ni, np)
phi_ = toPhi_(y, u, sign, no, ni, np);

== matlab function T_junction_mpc/SupervisoryController/paramEst1/Param Estimator (RLS)/RLS/MATLAB Function ==
  data: theta input; phi input; epsil input; EN input; p_ input; dPmod_ input; lambda input; dtheta output; P input; dP output; L output; no parameter; ni parameter; np parameter
function [dtheta, dP, L] = rls(theta, phi, epsil, EN, p_, dPmod_, lambda, P, no, ni, np)
[dtheta, dP, L] = rls_(theta, phi, epsil, EN, p_, dPmod_, lambda, P, no, ni, np);

== matlab function T_junction_mpc/SupervisoryController/paramEst2/Param Estimator (RLS)/RLS/MATLAB Function ==
  data: theta input; phi input; epsil input; EN input; p_ input; dPmod_ input; lambda input; dtheta output; P input; dP output; L output; no parameter; ni parameter; np parameter
function [dtheta, dP, L] = rls(theta, phi, epsil, EN, p_, dPmod_, lambda, P, no, ni, np)
[dtheta, dP, L] = rls_(theta, phi, epsil, EN, p_, dPmod_, lambda, P, no, ni, np);
